simulink model "Hybrid_Series"  (R2017b)
settings: Solver=VariableStepAuto  StartTime=0.0  StopTime=20  RelTol=1e-3  AbsTol=1e-3  EnableMultiTasking=on
model workspace (MATLAB code in the model file):
  | v0                 = 15; % Initial vehicle speed
  | wheel_radius = 0.3; % Wheel radius
  | k                   = 1e-2; % Motor losses (W/(N*M)^2)
  | t_torque        = 0.02; % Electric motor time constant
  | rpm0             = 2000; % Engine initial speed demand
values from neighbouring files (symbols this model uses):
  HEV_Param =     [DataWorkSpace.mat]
libraries: fl_lib x83, nesl_utility x27, sdl_lib x5, elec_lib x2
(part 1 of 2)
CloseFcn:
  | try,close(h1_sdl_hybrid_series),end
  | clear h1_sdl_hybrid_series
  | try,close(h2_sdl_hybrid_series),end
  | clear h2_sdl_hybrid_series
  | 
  | 
  | clear simlog_sdl_hybrid_series
Description:
  | Series Hybrid Transmission
  | 
  | Copyright 2008-2017 The MathWorks, Inc.
settings Model: FPTRunName=Active  Creator=MathWorks  LastModifiedBy=Charlie
settings DataIOCC: LimitDataPoints=on  MaxDataPoints=15000  SaveFormat=Array  SignalLoggingSaveFormat=ModelDataLogs  SignalLoggingName=logsout_sdl_hybrid_series
settings OptimizationCC: ExpressionDepthLimit=2147483647  LifeSpan=inf
settings DebuggingCC: UnderspecifiedInitializationDetection=Classic  MergeDetectMultiDrivingBlocksExec=none  FcnCallInpInsideContextMsg=warning  StateNameClashWarn=warning  SFUnexpectedBacktrackingDiag=warning  SFNoUnconditionalDefaultTransitionDiag=warning  SFExecutionAtInitializationDiag=none
settings HardwareCC: ProdBitPerPointer=32  ProdBitPerSizeT=32  ProdBitPerPtrDiffT=32  ProdLargestAtomicFloat=None  ProdIntDivRoundTo=Undefined  ProdEndianess=Unspecified  ProdWordSize=32  ProdHWDeviceType=32-bit Generic
settings ModelReferenceCC: PropagateSignalLabelsOutOfModel=off
settings CodeAppCC: StateflowObjectComments=on
settings GRTTargetCC: TargetLangStandard=C89/C90 (ANSI)  GeneratePreprocessorConditionals=Disable all  CombineOutputUpdateFcns=off  GRTInterface=on
settings ConfigComp: CovMetricSettings=dw  CovHtmlReporting=on  CovSaveCumulativeToWorkspaceVar=on  CovSaveSingleToWorkspaceVar=on  CovShowResultsExplorer=off  CovExternalEMLEnable=off
settings SimscapeCC: SimscapeLogType=all  SimscapeLogSimulationStatistics=on  SimscapeLogOpenViewer=on  SimscapeLogName=simlog_sdl_hybrid_series  SimscapeLogDataHistory=10000

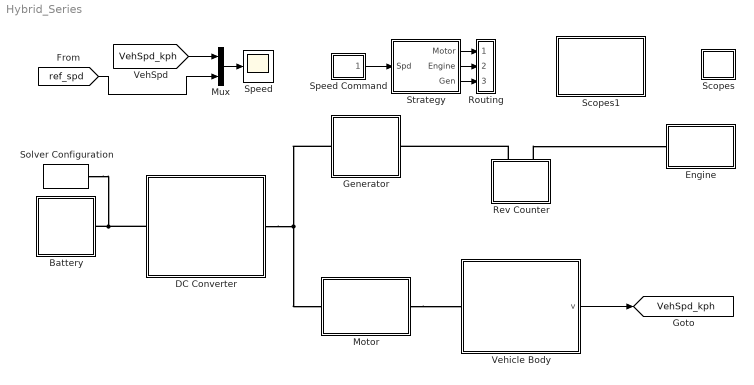
== system Hybrid_Series ==
  Battery : Subsystem
      mask Display:
      | % Plot points to set plot range
      | color('white');plot(1.5, 2.5);plot(-1.5, -2)
      | color('black');
      | % Battery icon
      | plot([0 0], [2.5 1.3])
      | plot([0 0], [-0.6 -1.6])
      | patch([-1 1 1 -1]*0.4, [1 1 -1 -1]*0.15+0.7,[0;0;0]);
      | patch([-1 1 1 -1]*0.4, [1 1 -1 -1]*0.15-0.6,[0;0;0]);
      | patch([-1 1 1 -1]*0.8, [1 1 -1 -1]*0.15+1.3,[0;0;0]);
      | patch([-1 1 1 -1]*0.8, [1 1 -1 -1]*0.15+0.0,[0;0;0]);
  DC Converter : Subsystem  mask{Vout=HEV_Param.DCDCConv.Output_Voltage, RLoadLoss=HEV_Param.DCDCConv.Resistance_Losses, Kp=HEV_Param.DCDCConv.Kp, Ki=HEV_Param.DCDCConv.Ki}
      mask prompts: Vout "Output Voltage (V)"; RLoadLoss "Resistance, Load Dependent Losses (Ohm)"; Kp "Proportional Gain"; Ki "Integral Gain"
      mask Display: image('D:\Matlab\Powertrain\Simscape\DC.jpg');
  Engine : Subsystem
      mask Display:
      | patch([0 374 374 0 0],[183 40 40 183 183],[1 1 1]);
      | plot([200.294537656123;201.704177092068;202.879954177142;203.81054553527;204.486989062962;204.902770239264;205.053884864158;204.938877621199;204.558856093007;203.917480094638;203.02092642757;201.877829393721;200.499197642409;198.898308151034;197.090578360535;195.093417696999;192.926059909376;191.349221415216], [79.0962651705123;81.4129472419303;83.856642682368;86.4038173688741;89.0299406167901;91.7097214236537;94.4173520353776;97.1267564890293;99.8118417386092;102.446748945347;105.006102512455;107.465254465996;109.80052182835;111.989414698229;114.010852840726;115.845368701499;117.475294889959;118.468271604945])
      | plot([180.070315486255;177.215173525063;174.340173090774;171.473002009205;168.641272705228;165.872256280019;163.192619875453;160.628169854943;158.203603274058;155.942270034374;153.865948011161;151.994633320535;150.346347745932;148.936965178479;147.780058742747;146.886770080143;146.265702048809;145.922835873396;145.861473542603;146.08220600922;146.58290749893;147.358755982674;148.402279615432;149.703428694174;151.249672441989;153.026119686324;155.015662269112;157.199139807684;159.555524219735;162.062122235246;164.694793945081;167.42818528151;170.23597219174;173.091114152932;175.966114587221;178.83328566879;181.665014972767;184.434031397976;185.486929355725], [123.25590763568;123.598773811093;123.660136141886;123.439403675268;122.938702185559;122.162853701815;121.119330069056;119.818180990315;118.2719372425;116.495489998164;114.505947415377;112.322469876805;109.966085464754;107.459487449243;104.826815739408;102.093424402979;99.2856374927491;96.4304955315569;93.5554950972677;90.688324015699;87.8565947117214;85.0875782865128;82.4079418819464;79.8434918614364;77.4189252805513;75.1575920408679;73.081270017655;71.2099553270291;69.5616697524256;68.1522871849724;66.9953807492411;66.1020920866371;65.4810240553025;65.1381578798894;65.0767955490969;65.2975280157144;65.7982295054238;66.5740779891678;66.9481130562871])
      | plot([182.088349247351;182.056804583223;181.962474383197;181.806267098667;181.589687091173;181.314820144583;180.98431337785;180.601349751811;180.169617415534;179.693274187426;179.176907513169;178.625490286111;178.044332955585;177.439032384376;176.815417947876;176.17949539401;175.537389004603;174.895282615196;174.25936006133;173.63574562483;173.030445053621;172.449287723095;171.897870496037;171.38150382178;170.905160593672;170.473428257395;170.090464631356;169.759957864623;169.485090918033;169.268510910539;169.112303626009;169.017973425983;168.986428761855;169.017973425983;169.112303626009;169.268510910539;169.485090918033;169.759957864623;170.090464631356;170.473428257395;170.905160593672;171.38150382178;171.897870496037;172.449287723095;173.030445053621;173.63574562483;174.25936006133;174.895282615196;175.537389004603;176.17949539401;176.815417947876;177.439032384376;178.044332955585;178.625490286111;179.176907513169;179.693274187426;180.169617415534;180.601349751811;180.98431337785;181.314820144583;181.589687091173;181.806267098667;181.962474383197;182.056804583223;182.088349247351;182.088349247351], [94.3432759959251;93.7073437064164;93.0775357924916;92.4599176486499;91.8604372752408;91.2848679959696;90.7387528576339;90.2273512475527;89.7555882427917;89.3280071789786;88.9487258954975;88.6213970784445;88.3491730832641;88.1346755758426;87.9799702844327;87.8865471055612;87.8553057555109;87.8865471055612;87.9799702844327;88.1346755758426;88.3491730832641;88.6213970784445;88.9487258954975;89.3280071789786;89.7555882427917;90.2273512475527;90.7387528576339;91.2848679959696;91.8604372752408;92.4599176486499;93.0775357924916;93.7073437064164;94.3432759959251;94.9792082854337;95.6090161993586;96.2266343432003;96.8261147166093;97.4016839958805;97.9477991342162;98.4592007442974;98.9309637490584;99.3585448128716;99.7378260963527;100.065154913406;100.337378908586;100.551876416008;100.706581707417;100.800004886289;100.831246236339;100.800004886289;100.706581707417;100.551876416008;100.337378908586;100.065154913406;99.7378260963526;99.3585448128716;98.9309637490584;98.4592007442974;97.9477991342162;97.4016839958805;96.8261147166093;96.2266343432003;95.6090161993586;94.9792082854338;94.3432759959251;94.3432759959251])
      | plot([201.615249970928;201.583705306799;201.489375106774;201.333167822243;201.11658781475;200.84172086816;200.511214101427;200.128250475388;199.69651813911;199.220174911002;198.703808236745;198.152391009688;197.571233679162;196.965933107953;196.342318671452;195.706396117586;195.06428972818;194.422183338773;193.786260784907;193.162646348407;192.557345777197;191.976188446671;191.424771219614;190.908404545357;190.432061317249;190.000328980971;189.617365354932;189.286858588199;189.011991641609;188.795411634116;188.639204349585;188.54487414956;188.513329485431;188.54487414956;188.639204349585;188.795411634116;189.011991641609;189.286858588199;189.617365354932;190.000328980971;190.432061317249;190.908404545357;191.424771219614;191.976188446671;192.557345777197;193.162646348407;193.786260784907;194.422183338773;195.06428972818;195.706396117586;196.342318671452;196.965933107953;197.571233679162;198.152391009688;198.703808236745;199.220174911002;199.69651813911;200.128250475388;200.511214101427;200.84172086816;201.11658781475;201.333167822243;201.489375106774;201.583705306799;201.615249970928;201.615249970928], [74.7533852700144;74.1174529805057;73.487645066581;72.8700269227392;72.2705465493302;71.694977270059;71.1488621317233;70.6374605216421;70.165697516881;69.7381164530679;69.3588351695868;69.0315063525339;68.7592823573535;68.5447848499319;68.390079558522;68.2966563796505;68.2654150296003;68.2966563796505;68.390079558522;68.5447848499319;68.7592823573535;69.0315063525339;69.3588351695868;69.7381164530679;70.165697516881;70.6374605216421;71.1488621317233;71.694977270059;72.2705465493302;72.8700269227392;73.487645066581;74.1174529805057;74.7533852700144;75.3893175595231;76.0191254734479;76.6367436172896;77.2362239906986;77.8117932699698;78.3579084083055;78.8693100183867;79.3410730231478;79.7686540869609;80.147935370442;80.4752641874949;80.7474881826754;80.9619856900969;81.1166909815068;81.2101141603783;81.2413555104285;81.2101141603783;81.1166909815068;80.9619856900969;80.7474881826753;80.4752641874949;80.147935370442;79.7686540869609;79.3410730231478;78.8693100183867;78.3579084083055;77.8117932699698;77.2362239906986;76.6367436172896;76.0191254734479;75.3893175595231;74.7533852700145;74.7533852700144])
      | plot([201.615249970928;201.583705306799;201.489375106774;201.333167822243;201.11658781475;200.84172086816;200.511214101427;200.128250475388;199.69651813911;199.220174911002;198.703808236745;198.152391009688;197.571233679162;196.965933107953;196.342318671452;195.706396117586;195.06428972818;194.422183338773;193.786260784907;193.162646348407;192.557345777197;191.976188446671;191.424771219614;190.908404545357;190.432061317249;190.000328980971;189.617365354932;189.286858588199;189.011991641609;188.795411634116;188.639204349585;188.54487414956;188.513329485431;188.54487414956;188.639204349585;188.795411634116;189.011991641609;189.286858588199;189.617365354932;190.000328980971;190.432061317249;190.908404545357;191.424771219614;191.976188446671;192.557345777197;193.162646348407;193.786260784907;194.422183338773;195.06428972818;195.706396117586;196.342318671452;196.965933107953;197.571233679162;198.152391009688;198.703808236745;199.220174911002;199.69651813911;200.128250475388;200.511214101427;200.84172086816;201.11658781475;201.333167822243;201.489375106774;201.583705306799;201.615249970928;201.615249970928], [74.7533852700144;74.1174529805057;73.487645066581;72.8700269227392;72.2705465493302;71.694977270059;71.1488621317233;70.6374605216421;70.165697516881;69.7381164530679;69.3588351695868;69.0315063525339;68.7592823573535;68.5447848499319;68.390079558522;68.2966563796505;68.2654150296003;68.2966563796505;68.390079558522;68.5447848499319;68.7592823573535;69.0315063525339;69.3588351695868;69.7381164530679;70.165697516881;70.6374605216421;71.1488621317233;71.694977270059;72.2705465493302;72.8700269227392;73.487645066581;74.1174529805057;74.7533852700144;75.3893175595231;76.0191254734479;76.6367436172896;77.2362239906986;77.8117932699698;78.3579084083055;78.8693100183867;79.3410730231478;79.7686540869609;80.147935370442;80.4752641874949;80.7474881826754;80.9619856900969;81.1166909815068;81.2101141603783;81.2413555104285;81.2101141603783;81.1166909815068;80.9619856900969;80.7474881826753;80.4752641874949;80.147935370442;79.7686540869609;79.3410730231478;78.8693100183867;78.3579084083055;77.8117932699698;77.2362239906986;76.6367436172896;76.0191254734479;75.3893175595231;74.7533852700145;74.7533852700144])
      | plot([142.90856779553;142.90856779553;208.103220211342;208.103220211342], [139.948037685826;218.181620584801;218.181620584801;139.948037685826])
      | plot([142.90856779553;208.103220211342], [179.064829135314;179.064829135314])
      | plot([149.459528038278;149.459528038278], [179.064829135314;172.576858894899])
      | plot([201.615249970928;201.615249970928], [179.064829135314;172.576858894899])
      | plot([142.90856779553;208.103220211342;208.103220211342;142.90856779553;142.90856779553], [179.064829135314;179.064829135314;152.986968168989;152.986968168989;179.064829135314])
      | plot([142.90856779553;208.103220211342], [192.103759618476;192.103759618476])
      | plot([180.639579193667;200.229469919577], [99.0045361686498;79.4776354450732])
      | plot([173.332738922909;192.92262964882], [87.8553057555109;68.3284050319344])
      | plot([183.663099305704;200.481429928914], [153.553878189996;76.9580353517085])
      | plot([184.544959338382;174.970478983596], [95.0361660216004;153.553878189996])
      | plot([183.474129298702;186.749609420076;206.654450157657;201.615249970928;197.961829835549], [76.9580353517085;62.0923948008567;67.8874750155956;88.1702557671815;87.7923157531768])
      | plot([164.199188584462;187.694459455088], [94.7842060122639;95.1621460262686])
      | plot([175.537389004603;175.285428995267], [106.50034644641;81.9342455361038])
      | plot([142.90856779553;208.103220211342], [172.576858894899;172.576858894899])
      | plot([297.86397353746;317.389525743201], [71.0999651346356;71.0999651346356]+60)
      | plot([269.518472487107;297.86397353746;297.86397353746;269.518472487107;269.518472487107], [85.2727156598121;85.2727156598121;56.927214609459;56.927214609459;85.2727156598121]+60)
      | plot([258.180272066966;269.518472487107;269.518472487107;258.180272066966], [42.7544640842825;42.7544640842825;99.4454661849886;99.4454661849886]+60)
      | plot([108.893966535106;108.245686045801;107.603648851995;106.974038122836;106.362917353826;105.776171972045;105.219452656266;104.698120917834;104.217197466378;103.781313857637;103.394667889039;103.060983172626;102.783473274627;102.564810767061;102.40710148941;102.31186426823;102.280016290024;102.280016290024;102.31186426823;102.40710148941;102.564810767061;102.783473274627;103.060983172626;103.394667889039;103.781313857637;104.217197466378;104.698120917834;105.219452656266;105.776171972045;106.362917353826;106.974038122836;107.603648851995;108.245686045801;108.893966535106;249.67662175186;250.324902241165;250.966939434972;251.596550164131;252.20767093314;252.794416314921;253.3511356307;253.872467369133;254.353390820588;254.78927442933;255.175920397927;255.50960511434;255.787115012339;256.005777519905;256.163486797556;256.258724018736;256.290571996942;256.290571996942;256.258724018736;256.163486797556;256.005777519905;255.787115012339;255.50960511434;255.175920397927;254.78927442933;254.353390820588;253.872467369133;253.3511356307;252.794416314921;252.20767093314;251.596550164131;250.966939434972;250.324902241165;249.67662175186;108.893966535106], [233.173241140321;233.141393162114;233.046155940935;232.888446663284;232.669784155718;232.392274257719;232.058589541306;231.671943572708;231.236059963967;230.755136512511;230.233804774079;229.6770854583;229.090340076519;228.479219307509;227.84960857835;227.207571384544;226.559290895239;46.5338642243296;45.8855837350246;45.2435465412178;44.6139358120588;44.0028150430496;43.4160696612682;42.8593503454891;42.3380186070568;41.8570951556014;41.4212115468599;41.0345655782626;40.7008808618494;40.42337096385;40.2047084562844;40.0469991786335;39.9517619574538;39.9199139792472;39.9199139792472;39.9517619574538;40.0469991786335;40.2047084562844;40.42337096385;40.7008808618494;41.0345655782626;41.4212115468599;41.8570951556014;42.3380186070568;42.8593503454891;43.4160696612682;44.0028150430496;44.6139358120588;45.2435465412178;45.8855837350246;46.5338642243296;226.559290895239;227.207571384544;227.84960857835;228.479219307509;229.090340076519;229.6770854583;230.233804774079;230.755136512511;231.236059963967;231.671943572708;232.058589541306;232.392274257719;232.669784155718;232.888446663284;233.046155940935;233.141393162114;233.173241140321;233.173241140321])
  Generator : Subsystem
      mask Display: image('D:\Matlab\Powertrain\Simscape\Yanan_400_hertz_brushless_generator_alternator_3984_3.jpg');
  Motor : Subsystem
      mask Display: image('D:\Matlab\Powertrain\Simscape\IM2014100062CO_300dpi.jpg');
  Mux : Mux  Inputs=2
  Rev Counter : Subsystem
      mask Display: image('D:\Matlab\Powertrain\Simscape\Rev-counter.jpg');
  Routing : Subsystem
  Scopes : Subsystem
  Scopes1 : Subsystem  mask(Data Acquisition){}
      mask Display: image('D:\Matlab\Powertrain\Plot\Fuel_Tank.jpg');
  Solver Configuration : nesl_utility/Solver Configuration  PhysicalDomain=network_engine_domain  SubClassName=solver  LeftPortType=input  RightPortType=generic  Accelerate=off  Tones=[]  Harmonics=[]  SimulateNoise=off  Profile=off  UseLocalSampling=off  EnableSwitchedLinearOptims=on  FrequencyDomain=off  UseCCode=off  RelTol=0.001  AbsTol=1e-06  MinStep=1e-09  ToWorkspace=off  RevertToSquareIcSolve=off  NumHomotopyIterations=100  PhasorMode=off  PhasorModeNumHarmonics=1  DoDC=off  ResidualTolerance=1e-9  UseLocalSolver=off  LocalSolverChoice=NE_BACKWARD_EULER_ADVANCER  LocalSolverSampleTime=0.005  DoFixedCost=off  MaxNonlinIter=3  MaxModeIter=2  LinearAlgebra=Sparse  DelaysMemoryBudget=1024  AutomaticFiltering=on  FilteringTimeConstant=0.001
  Speed : Scope
  Speed Command : Subsystem
  Strategy : Subsystem
  Vehicle Body : Subsystem
      mask Display: image('D:\Matlab\Powertrain\Simscape\smart_fortw.jpg');
  tag scope: VehSpd_kph=global
  wires:
  Speed Command/1(Spd) -> Strategy/1(Spd)
  Strategy/1(Motor) -> Routing/1(M)
  Strategy/2(Engine) -> Routing/2(E)
  Strategy/3(Gen) -> Routing/3(G)
  Mux/1 -> Speed/1
  [ref_spd] -> Mux/2
  Vehicle Body/1(v) -> [VehSpd_kph]
  [VehSpd_kph] -> Mux/1
  connections:
  Motor/LConn1 -- Vehicle Body/LConn1
  Generator/RConn1 -- DC Converter/RConn1 -- Motor/RConn1
  Solver Configuration/RConn1 -- DC Converter/LConn1 -- Battery/LConn1
  Rev Counter/LConn2 -- Engine/RConn1
  Rev Counter/LConn1 -- Generator/LConn1

== system Hybrid_Series/Battery ==
  Calculations : Subsystem
  Current Sensor : fl_lib/Electrical/Electrical Sensors/Current Sensor
  DC Voltage Source : fl_lib/Electrical/Electrical Sources/DC Voltage Source  v0=201.6 V
  Electrical Reference : fl_lib/Electrical/Electrical Elements/Electrical Reference
  Internal Resistance : fl_lib/Electrical/Electrical Elements/Resistor  R=0.05 Ohm  i_specify=off  i_priority=High  i=0 A  i_nominal_specify=off  i_nominal_unit=A  i_nominal_value=1  v_specify=off  v_priority=High  v=0 V  v_nominal_specify=off  v_nominal_unit=V  v_nominal_value=1
  Voltage Sensor : fl_lib/Electrical/Electrical Sensors/Voltage Sensor
  V : PMIOPort  Port=1  Side=Left
  connections:
  DC Voltage Source/LConn1 -- Internal Resistance/LConn1
  Internal Resistance/RConn1 -- V/RConn1 -- Voltage Sensor/LConn1
  Current Sensor/RConn2 -- DC Voltage Source/RConn1
  Voltage Sensor/RConn1 -- Calculations/LConn1
  Current Sensor/RConn1 -- Calculations/LConn2
  Electrical Reference/LConn1 -- Current Sensor/LConn1 -- Voltage Sensor/RConn2

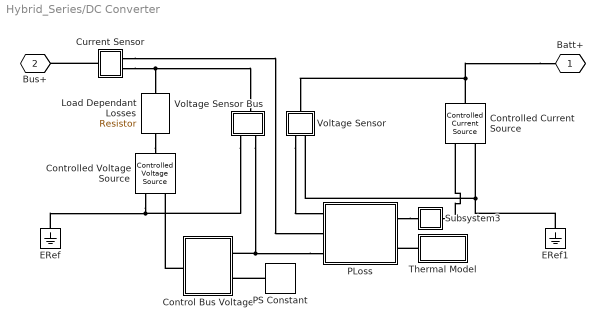
== system Hybrid_Series/DC Converter ==
  Control Bus Voltage : Subsystem
  Controlled Current Source : fl_lib/Electrical/Electrical Sources/Controlled Current Source
  Controlled Voltage Source : fl_lib/Electrical/Electrical Sources/Controlled Voltage Source
  Current Sensor : Subsystem
  ERef : fl_lib/Electrical/Electrical Elements/Electrical Reference
  ERef1 : fl_lib/Electrical/Electrical Elements/Electrical Reference
  Load Dependant Losses : fl_lib/Electrical/Electrical Elements/Resistor  R=RLoadLoss Ohm  i_specify=off  i_priority=High  i=0 A  i_nominal_specify=off  i_nominal_unit=A  i_nominal_value=1  v_specify=off  v_priority=High  v=0 V  v_nominal_specify=off  v_nominal_unit=V  v_nominal_value=1
  PLoss : Subsystem
  PS Constant : fl_lib/Physical Signals/Sources/PS Constant  constant=Vout
  Subsystem3 : Subsystem
      mask Display: disp('S')
  Thermal Model : Subsystem
  Voltage Sensor : Subsystem
  Voltage Sensor Bus : Subsystem
  " Batt+" : PMIOPort  Tag=PMCPort  Port=1  Side=Left
  " Bus+" : PMIOPort  Tag=PMCPort  Port=2  Side=Right
  connections:
  Thermal Model/LConn1 -- PLoss/RConn2
  PLoss/LConn3 -- Control Bus Voltage/LConn1 -- Voltage Sensor Bus/RConn2
  Subsystem3/LConn1 -- Controlled Current Source/RConn1
  PS Constant/RConn1 -- Control Bus Voltage/LConn2
  Control Bus Voltage/RConn1 -- Controlled Voltage Source/RConn1
  " Batt+"/RConn1 -- Controlled Current Source/LConn1 -- Voltage Sensor/LConn1
  Controlled Current Source/RConn2 -- ERef1/LConn1 -- Voltage Sensor/RConn2
  Load Dependant Losses/RConn1 -- Controlled Voltage Source/LConn1
  Controlled Voltage Source/RConn2 -- ERef/LConn1 -- Voltage Sensor Bus/RConn1
  Current Sensor/LConn1 -- " Bus+"/RConn1
  Current Sensor/RConn2 -- Load Dependant Losses/LConn1 -- Voltage Sensor Bus/LConn1
  Voltage Sensor/RConn1 -- PLoss/LConn1
  Current Sensor/RConn1 -- PLoss/LConn2
  PLoss/RConn1 -- Subsystem3/RConn1

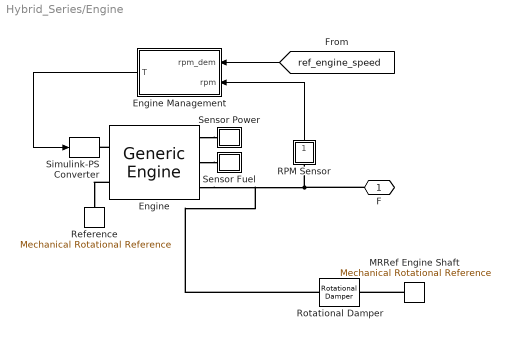
== system Hybrid_Series/Engine ==
  Engine : sdl_lib/Engines/Generic Engine  model_parameterization=1  engine_type=1  P_max=52 kW  w_P_max=6000 rpm  w_max=7000 rpm  w_min=500 rpm  w_tab=[ 500 1000 2e+3 3e+3 4e+3 5e+3 6e+3 7e+3 ] rpm  trq_tab=[ 40 41 42 46 49 42 41 40 ] N*m  pwr_tab=[ 2e+4 4e+4 7.8e+4 1.2e+5 1.45e+5 1.48e+5 1.25e+5 6e+4 ] W  interp_method=1  model_inertia=1  inertia=HEV_Param.ICE.Shaft_Inertia kg*m^2  initial_velocity=2000 rpm  model_time_constant=1  time_constant=0.4 s  T0=0  w_thr=100 rpm  idle_speed=1  idle_speed_reference=800 rpm  tau_controller=1 s  idle_w_thr=1 rpm  redline=0  redline_speed=7000 rpm  tau_redline=1 s  redline_w_thr=1 rpm  fc_model=1  fc_per_rev=6.2 mg/rev  displaced_volume=400 cm^3  rev_per_cycle=2  fc_w_tab=[ 1000 2e+3 3e+3 4e+3 5e+3 6e+3 ] rpm  fc_trq_tab=[ 0 80 160 200 240 320 360 400 ] N*m  fc_tab=[ 0.5 0.9 1.4 1.6 1.9 2.7 3.4 4.4; 1 1.7 2.7 3.1 3.6 5 6 7.4; 1.4 2.7 4 4.8 5.6 7.5 8.5 10.5; 2 3.6 5.8 6.7 8 10.4 11.7 13.3; 2.5 4.8 7.9 9.4 10.8 14 16.2 18.6; 3.1 6 10.3 11.9 13.8 18.4 22 26.5 ] g/s  bmep_tab=[ 0 250 500 625 750 1000 1.15e+3 1.25e+3 ] kPa  bsfc_tab=[ 410 380 300 280 270 290 320 380; 410 370 290 270 260 270 285 320; 415 380 290 275 265 270 270 300; 420 390 310 290 285 280 280 285; 430 410 340 320 310 300 310 320; 450 430 370 340 330 330 350 380 ] g/hr/kW  fc_interp_method=1
      settings: SourceProductName=Simscape Driveline  SourceProductBaseCode=LD
  Engine Management : Subsystem
  MRRef Engine Shaft : fl_lib/Mechanical/Rotational Elements/Mechanical Rotational Reference
  RPM Sensor : Subsystem
      mask Display: disp('S');
  Reference : fl_lib/Mechanical/Rotational Elements/Mechanical Rotational Reference
  Rotational Damper : fl_lib/Mechanical/Rotational Elements/Rotational Damper  D=HEV_Param.ICE.Friction N*m/(rad/s)  w_specify=off  w_priority=High  w=0 rad/s  w_nominal_specify=off  w_nominal_unit=rad/s  w_nominal_value=1  t_specify=off  t_priority=High  t=0 N*m  t_nominal_specify=off  t_nominal_unit=N*m  t_nominal_value=1
  Sensor Fuel : Subsystem
  Sensor Power : Subsystem
  Simulink-PS Converter : nesl_utility/Simulink-PS Converter  PhysicalDomain=network_engine_domain  SubClassName=ps_input  LeftPortType=input  RightPortType=output  PseudoPeriodic=off  Frequencies=[]  NoiseDistribution=none  NoiseParameters=[]  Unit=1  AffineConversion=off  FilteringAndDerivatives=zero  SimscapeFilterOrder=1  InputFilterTimeConstant=.001  UdotUserProvided=0
  F : PMIOPort  Port=1  Side=Right
  wires:
  RPM Sensor/1(rpm) -> Engine Management/2(rpm)
  [ref_engine_speed] -> Engine Management/1(rpm_dem)
  Engine Management/1(T) -> Simulink-PS Converter/1
  connections:
  F/RConn1 -- Rotational Damper/LConn1 -- Engine/RConn3 -- RPM Sensor/LConn1
  Engine/LConn2 -- Reference/LConn1
  Engine/LConn1 -- Simulink-PS Converter/RConn1
  Engine/RConn1 -- Sensor Power/LConn1
  Engine/RConn2 -- Sensor Fuel/LConn1
  MRRef Engine Shaft/LConn1 -- Rotational Damper/RConn1

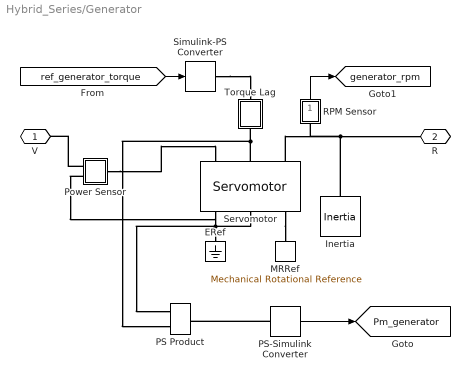
== system Hybrid_Series/Generator ==
  ERef : fl_lib/Electrical/Electrical Elements/Electrical Reference
  Inertia : fl_lib/Mechanical/Rotational Elements/Inertia  inertia=HEV_Param.Generator.Shaft_Inertia kg*m^2  w_specify=on  w_priority=High  w=0 rad/s  w_nominal_specify=off  w_nominal_unit=rad/s  w_nominal_value=1  t_specify=off  t_priority=High  t=0 N*m  t_nominal_specify=off  t_nominal_unit=N*m  t_nominal_value=1
  MRRef : fl_lib/Mechanical/Rotational Elements/Mechanical Rotational Reference
  PS Product : fl_lib/Physical Signals/Functions/PS Product
      settings: SourceProductName=Simscape
  PS-Simulink Converter : nesl_utility/PS-Simulink Converter  PhysicalDomain=network_engine_domain  SubClassName=ps_output  LeftPortType=input  RightPortType=output  PseudoPeriodic=off  Frequencies=[]  Unit=1  AffineConversion=off
  Power Sensor : Subsystem  AncestorBlock=HEV_Electrical_Lib/System Level/Synchronous Generator & Drive/Power Sensor
      mask Display: disp('S')
  RPM Sensor : Subsystem
      mask Display: disp('S')
  Servomotor : elec_lib/Actuators & Drivers/Rotational Actuators/Servomotor  torque_speed_param=1  w_t=HEV_Param.Generator.TorqSpdLUT.SpeedRPM rpm  T_t=HEV_Param.Generator.TorqSpdLUT.TorqueNm N*m  torque_max=0.1 N*m  power_max=30 W  Tc=HEV_Param.Generator.TorqueControl_TimeConst s  losses_param=1  eff=90  w_eff=2000 rpm  T_eff=200 N*m  Piron=0 W  Pbase=HEV_Param.Generator.TorqIndep_Elec_Loss W  w_eff_vec=[-8000 -4000 0 4000 8000] rpm  T_eff_vec=[0 0.03 0.06 0.09] N*m  losses_mat=[1.49 1.67 2.21 3.10; 0.42 0.69 1.14 2.03; 0.06 0.24 0.78 1.68; 0.42 0.69 1.14 2.03; 1.49 1.67 2.21 3.10] W  efficiency_mat=[95 95 95 95; 95 95 95 95; 95 95 95 95; 95 95 95 95; 95 95 95 95]  Res=HEV_Param.Generator.Series_Resistance Ohm  J=0 kg*m^2  lam=HEV_Param.Generator.Damping N*m/(rad/s)  speed0=0 rpm  faulted_specify=off  faulted_priority=None  faulted=0  faulted_nominal_specify=off  faulted_nominal_unit=1  faulted_nominal_value=1  alpha=0.00393 1/K  Tmeas=25 degC  Tmeas2=125 degC  losses_mat_T2=[1.49 1.74 2.49 3.74;0.42 0.67 1.42 2.67;0.06 0.31 1.06 2.31;0.42 0.67 1.42 2.67;1.49 1.74 2.49 3.74] W  efficiency_mat_T2=[95 95 95 95; 95 95 95 95; 95 95 95 95; 95 95 95 95; 95 95 95 95]  thermal_mass=100 J/K  initial_temperature=25 degC  fault_condition=1  fault_threshold=0.5
      settings: SourceProductName=Simscape Electronics  SourceProductBaseCode=SN
  Simulink-PS Converter : nesl_utility/Simulink-PS Converter  PhysicalDomain=network_engine_domain  SubClassName=ps_input  LeftPortType=input  RightPortType=output  PseudoPeriodic=off  Frequencies=[]  NoiseDistribution=none  NoiseParameters=[]  Unit=N*m  AffineConversion=off  FilteringAndDerivatives=zero  SimscapeFilterOrder=1  InputFilterTimeConstant=.001  UdotUserProvided=0
  Torque Lag : Subsystem
  V : PMIOPort  Port=1  Side=Right
  R : PMIOPort  Port=2  Side=Left
  tag scope: Pm_generator=global, generator_rpm=global
  wires:
  [ref_generator_torque] -> Simulink-PS Converter/1
  RPM Sensor/1(rpm) -> [generator_rpm]
  PS-Simulink Converter/1 -> [Pm_generator]
  connections:
  Servomotor/RConn1 -- Power Sensor/LConn2 -- ERef/LConn1
  Servomotor/RConn3 -- MRRef/LConn1
  Servomotor/LConn3 -- RPM Sensor/LConn1 -- Inertia/LConn1 -- R/RConn1
  Simulink-PS Converter/RConn1 -- Torque Lag/LConn1
  Torque Lag/RConn1 -- Servomotor/LConn2 -- PS Product/LConn2
  Servomotor/RConn2 -- PS Product/LConn1
  PS-Simulink Converter/LConn1 -- PS Product/RConn1
  Power Sensor/LConn1 -- V/RConn1
  Power Sensor/RConn1 -- Servomotor/LConn1

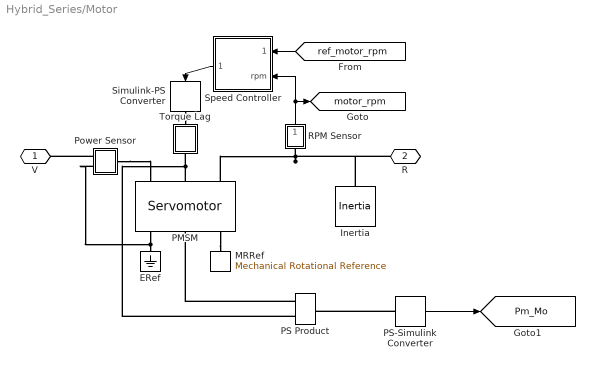
== system Hybrid_Series/Motor ==
  ERef : fl_lib/Electrical/Electrical Elements/Electrical Reference
  Inertia : fl_lib/Mechanical/Rotational Elements/Inertia  inertia=HEV_Param.Motor.Shaft_Inertia kg*m^2  w_specify=on  w_priority=High  w=0 rad/s  w_nominal_specify=off  w_nominal_unit=rad/s  w_nominal_value=1  t_specify=off  t_priority=High  t=0 N*m  t_nominal_specify=off  t_nominal_unit=N*m  t_nominal_value=1
  MRRef : fl_lib/Mechanical/Rotational Elements/Mechanical Rotational Reference
  PMSM : elec_lib/Actuators & Drivers/Rotational Actuators/Servomotor  torque_speed_param=1  w_t=HEV_Param.Motor.TorqSpdLUT.SpeedRPM rpm  T_t=HEV_Param.Motor.TorqSpdLUT.TorqueNm N*m  torque_max=0.1 N*m  power_max=30 W  Tc=HEV_Param.Motor.TorqueControl_TimeConst s  losses_param=1  eff=HEV_Param.Motor.Efficiency  w_eff=2000 rpm  T_eff=200 N*m  Piron=0 W  Pbase=0 W  w_eff_vec=[-8000 -4000 0 4000 8000] rpm  T_eff_vec=[0 0.03 0.06 0.09] N*m  losses_mat=[1.49 1.67 2.21 3.10; 0.42 0.69 1.14 2.03; 0.06 0.24 0.78 1.68; 0.42 0.69 1.14 2.03; 1.49 1.67 2.21 3.10] W  efficiency_mat=[95 95 95 95; 95 95 95 95; 95 95 95 95; 95 95 95 95; 95 95 95 95]  Res=HEV_Param.Motor.Series_Resistance Ohm  J=0 kg*m^2  lam=HEV_Param.Motor.Damping N*m/(rad/s)  speed0=0 rpm  faulted_specify=off  faulted_priority=None  faulted=0  faulted_nominal_specify=off  faulted_nominal_unit=1  faulted_nominal_value=1  alpha=0.00393 1/K  Tmeas=25 degC  Tmeas2=125 degC  losses_mat_T2=[1.49 1.74 2.49 3.74;0.42 0.67 1.42 2.67;0.06 0.31 1.06 2.31;0.42 0.67 1.42 2.67;1.49 1.74 2.49 3.74] W  efficiency_mat_T2=[95 95 95 95; 95 95 95 95; 95 95 95 95; 95 95 95 95; 95 95 95 95]  thermal_mass=100 J/K  initial_temperature=25 degC  fault_condition=1  fault_threshold=0.5
      settings: SourceProductName=Simscape Electronics  SourceProductBaseCode=SN
  PS Product : fl_lib/Physical Signals/Functions/PS Product
      settings: SourceProductName=Simscape
  PS-Simulink Converter : nesl_utility/PS-Simulink Converter  PhysicalDomain=network_engine_domain  SubClassName=ps_output  LeftPortType=input  RightPortType=output  PseudoPeriodic=off  Frequencies=[]  Unit=1  AffineConversion=off
  Power Sensor : Subsystem  AncestorBlock=HEV_Electrical_Lib/System Level/Synchronous Generator & Drive/Power Sensor
      mask Display: disp('S')
  RPM Sensor : Subsystem
      mask Display: disp('S')
  Simulink-PS Converter : nesl_utility/Simulink-PS Converter  PhysicalDomain=network_engine_domain  SubClassName=ps_input  LeftPortType=input  RightPortType=output  PseudoPeriodic=off  Frequencies=[]  NoiseDistribution=none  NoiseParameters=[]  Unit=N*m  AffineConversion=off  FilteringAndDerivatives=zero  SimscapeFilterOrder=1  InputFilterTimeConstant=.001  UdotUserProvided=0
  Speed Controller : Subsystem
  Torque Lag : Subsystem
  V : PMIOPort  Port=1  Side=Right
  R : PMIOPort  Port=2  Side=Left
  tag scope: Pm_Mo=global, motor_rpm=global
  wires:
  Speed Controller/1(T_ref) -> Simulink-PS Converter/1
  [ref_motor_rpm] -> Speed Controller/1(rpm_ref)
  RPM Sensor/1(rpm) -> [motor_rpm], Speed Controller/2(rpm)
  PS-Simulink Converter/1 -> [Pm_Mo]
  connections:
  RPM Sensor/LConn1 -- Inertia/LConn1 -- R/RConn1 -- PMSM/LConn3
  PMSM/LConn2 -- PS Product/LConn2 -- Torque Lag/RConn1
  PMSM/RConn1 -- Power Sensor/LConn2 -- ERef/LConn1
  PMSM/RConn3 -- MRRef/LConn1
  Simulink-PS Converter/RConn1 -- Torque Lag/LConn1
  PS-Simulink Converter/LConn1 -- PS Product/RConn1
  PS Product/LConn1 -- PMSM/RConn2
  Power Sensor/LConn1 -- V/RConn1
  Power Sensor/RConn1 -- PMSM/LConn1

== system Hybrid_Series/Rev Counter ==
  Gain : Gain  Gain=-1
  Ideal Rotational Motion Sensor : fl_lib/Mechanical/Mechanical Sensors/Ideal Rotational Motion Sensor  offset=0 rad
  Ideal Torque Sensor : fl_lib/Mechanical/Mechanical Sensors/Ideal Torque Sensor
  Mechanical Rotational Reference : fl_lib/Mechanical/Rotational Elements/Mechanical Rotational Reference
  PS-Simulink Converter : nesl_utility/PS-Simulink Converter  PhysicalDomain=network_engine_domain  SubClassName=ps_output  LeftPortType=input  RightPortType=output  PseudoPeriodic=off  Frequencies=[]  Unit=rpm  AffineConversion=off
  PS-Simulink Converter1 : nesl_utility/PS-Simulink Converter  PhysicalDomain=network_engine_domain  SubClassName=ps_output  LeftPortType=input  RightPortType=output  PseudoPeriodic=off  Frequencies=[]  Unit=N*m  AffineConversion=off
  A : PMIOPort  Port=1  Side=Left
  B : PMIOPort  Port=2  Side=Left
  tag scope: Carrier_Trq_Nm=global, EngSpd_RPM=global
  wires:
  PS-Simulink Converter/1 -> [EngSpd_RPM]
  PS-Simulink Converter1/1 -> Gain/1
  Gain/1 -> [Carrier_Trq_Nm]
  connections:
  PS-Simulink Converter/LConn1 -- Ideal Rotational Motion Sensor/RConn2
  Mechanical Rotational Reference/LConn1 -- Ideal Rotational Motion Sensor/RConn1
  Ideal Rotational Motion Sensor/LConn1 -- A/RConn1 -- Ideal Torque Sensor/LConn1
  Ideal Torque Sensor/RConn2 -- PS-Simulink Converter1/LConn1
  B/RConn1 -- Ideal Torque Sensor/RConn1

== system Hybrid_Series/Routing ==
  M : Inport
  E : Inport  Port=2
  G : Inport  Port=3
  tag scope: ref_engine_speed=global, ref_generator_torque=global, ref_motor_rpm=global
  wires:
  E/1 -> [ref_engine_speed]
  G/1 -> [ref_generator_torque]
  M/1 -> [ref_motor_rpm]

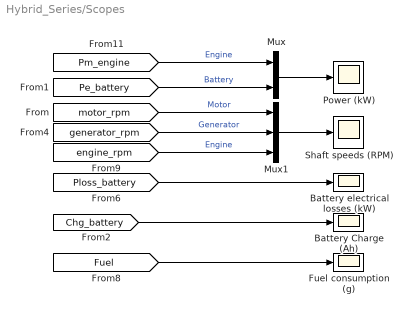
== system Hybrid_Series/Scopes ==
  Battery Charge (Ah) : Scope
  Battery electrical losses (kW) : Scope
  Fuel consumption (g) : Scope
  Mux : Mux  Inputs=2
  Mux1 : Mux  Inputs=3
  Power (kW) : Scope
  Shaft speeds (RPM) : Scope
  wires:
  Mux/1 -> Power (kW)/1
  Mux1/1 -> Shaft speeds (RPM)/1
  [motor_rpm] -> Mux1/1  "Motor"
  [generator_rpm] -> Mux1/2  "Generator"
  [engine_rpm] -> Mux1/3  "Engine"
  [Pm_engine] -> Mux/1  "Engine"
  [Pe_battery] -> Mux/2  "Battery"
  [Ploss_battery] -> Battery electrical losses (kW)/1
  [Fuel] -> Fuel consumption (g)/1
  [Chg_battery] -> Battery Charge (Ah)/1

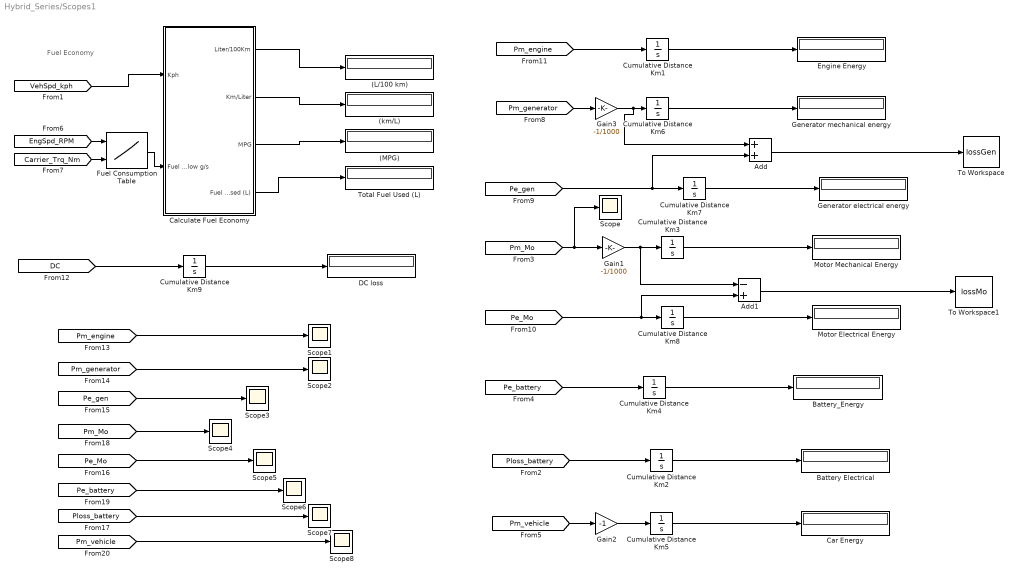
== system Hybrid_Series/Scopes1 ==
  note: Fuel Economy
  (L/100 km) : Display
      settings: Decimation=decimation
  (MPG) : Display
      settings: Decimation=decimation
  (km/L) : Display
      settings: Decimation=decimation
  Add : Sum
  Add1 : Sum  Inputs=-+
  Battery Electrical : Display
      settings: Decimation=decimation
  Battery_Energy : Display
      settings: Decimation=decimation
  Calculate Fuel Economy : Subsystem
  Car Energy : Display
      settings: Decimation=decimation
  Cumulative Distance Km{1..9} (9 alike) : Integrator  InitialCondition=eps
  DC loss : Display
      settings: Decimation=decimation
  Engine Energy : Display
      settings: Decimation=decimation
  Fuel Consumption Table : Lookup2D  RowIndex=HEV_Param.ICE.FC.Speed_Vector  ColumnIndex=HEV_Param.ICE.FC.Torque_Vector  Table=HEV_Param.ICE.FC.Consumption_Table
  Gain1 : Gain  Gain=-1/1000
  Gain2 : Gain  Gain=-1
  Gain3 : Gain  Gain=-1/1000
  Generator electrical energy : Display
      settings: Decimation=decimation
  Generator mechanical energy : Display
      settings: Decimation=decimation
  Motor Electrical Energy : Display
      settings: Decimation=decimation
  Motor Mechanical Energy : Display
      settings: Decimation=decimation
  Scope{,1..8} (9 alike) : Scope
  To Workspace : ToWorkspace  VariableName=lossGen  SampleTime=-1
      settings: Save2DSignal=2-D array (concatenate along first dimension)
  To Workspace1 : ToWorkspace  VariableName=lossMo  SampleTime=-1
      settings: Save2DSignal=2-D array (concatenate along first dimension)
  Total Fuel Used (L) : Display
      settings: Decimation=decimation
  wires:
  Cumulative Distance Km2/1 -> Battery Electrical/1
  [Ploss_battery] -> Cumulative Distance Km2/1
  Fuel Consumption Table/1 -> Calculate Fuel Economy/2(Fuel Flow g/s)
  Cumulative Distance Km5/1 -> Car Energy/1
  Gain2/1 -> Cumulative Distance Km5/1
  Cumulative Distance Km1/1 -> Engine Energy/1
  [Pm_engine] -> Cumulative Distance Km1/1
  Calculate Fuel Economy/1(Liter/100Km) -> (L/100 km)/1
  [VehSpd_kph] -> Calculate Fuel Economy/1(Kph)
  [Pe_battery] -> Cumulative Distance Km4/1
  [EngSpd_RPM] -> Fuel Consumption Table/1
  [Pm_Mo] -> Scope/1, Gain1/1
  Calculate Fuel Economy/3(MPG) -> (MPG)/1
  Cumulative Distance Km3/1 -> Motor Mechanical Energy/1
  [Carrier_Trq_Nm] -> Fuel Consumption Table/2
  Cumulative Distance Km4/1 -> Battery_Energy/1
  Calculate Fuel Economy/2(Km/Liter) -> (km/L)/1
  Calculate Fuel Economy/4(Fuel Used (L)) -> Total Fuel Used (L)/1
  [Pm_vehicle] -> Gain2/1
  Cumulative Distance Km6/1 -> Generator mechanical energy/1
  [Pm_generator] -> Gain3/1
  Gain3/1 -> Add/1, Cumulative Distance Km6/1
  [Pe_gen] -> Add/2, Cumulative Distance Km7/1
  Cumulative Distance Km7/1 -> Generator electrical energy/1
  Add/1 -> To Workspace/1
  Cumulative Distance Km8/1 -> Motor Electrical Energy/1
  Add1/1 -> To Workspace1/1
  [Pe_Mo] -> Add1/2, Cumulative Distance Km8/1
  Gain1/1 -> Add1/1, Cumulative Distance Km3/1
  Cumulative Distance Km9/1 -> DC loss/1
  [DC] -> Cumulative Distance Km9/1
  [Pm_engine] -> Scope1/1
  [Pm_generator] -> Scope2/1
  [Pe_gen] -> Scope3/1
  [Pm_Mo] -> Scope4/1
  [Pe_Mo] -> Scope5/1
  [Pe_battery] -> Scope6/1
  [Ploss_battery] -> Scope7/1
  [Pm_vehicle] -> Scope8/1

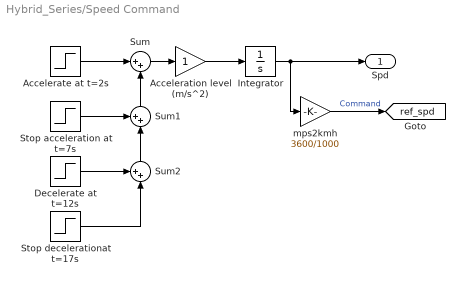
== system Hybrid_Series/Speed Command ==
  Accelerate at t=2s : Step  Time=2  SampleTime=0
  Acceleration level (m/s^2) : Gain
  Decelerate at t=12s : Step  Time=12  After=-1  SampleTime=0
  Integrator : Integrator  InitialCondition=v0
  Stop acceleration at t=7s : Step  Time=7  After=-1  SampleTime=0
  Stop decelerationat t=17s : Step  Time=17  SampleTime=0
  Sum : Sum  Inputs=|++
  Sum1 : Sum  Inputs=++|
  Sum2 : Sum  Inputs=++|
  mps2kmh : Gain  Gain=3600/1000
  Spd : Outport
  tag scope: ref_spd=global
  wires:
  mps2kmh/1 -> [ref_spd]  "Command"
  Stop decelerationat t=17s/1 -> Sum2/2
  Decelerate at t=12s/1 -> Sum2/1
  Acceleration level (m/s^2)/1 -> Integrator/1
  Sum2/1 -> Sum1/2
  Sum1/1 -> Sum/2
  Stop acceleration at t=7s/1 -> Sum1/1
  Integrator/1 -> Spd/1, mps2kmh/1
  Sum/1 -> Acceleration level (m/s^2)/1
  Accelerate at t=2s/1 -> Sum/1

== system Hybrid_Series/Strategy ==
  note: Generator torque demand has been set so that at the starting condition
      | the combustion engine is providing just enough power to keep the vehicle
      | moving at constant speed, and hence battery power is close to zero. The
      | engine RPM demand is set to 2000 rpm for good efficiency.
  Spd : Inport
  Convert to wheel RPM : Gain  Gain=60/(2*pi)/wheel_radius
  Engine RPM demand : Constant  Value=rpm0
  Generator torque demand : Constant  Value=-11
  Steady-state correction factor as proportional-only control : Gain  Gain=1.08
  Motor : Outport
  Engine : Outport  Port=2
  Gen : Outport  Port=3
  wires:
  Engine RPM demand/1 -> Steady-state correction factor as proportional-only control/1
  Spd/1 -> Convert to wheel RPM/1
  Convert to wheel RPM/1 -> Motor/1
  Steady-state correction factor as proportional-only control/1 -> Engine/1
  Generator torque demand/1 -> Gen/1

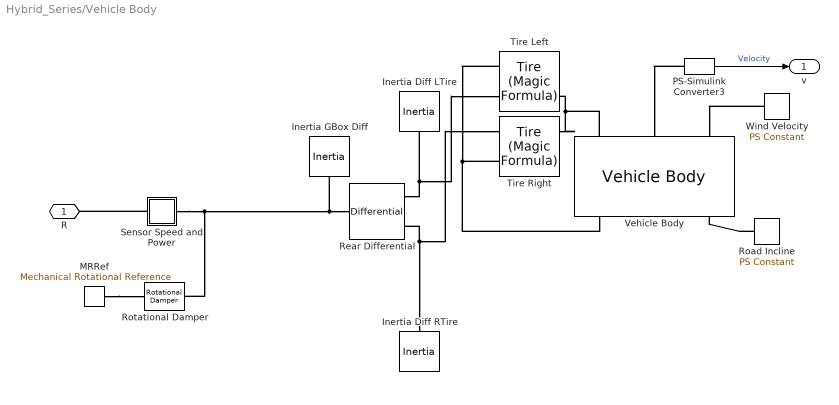
== system Hybrid_Series/Vehicle Body ==
  Inertia Diff LTire : fl_lib/Mechanical/Rotational Elements/Inertia  inertia=HEV_Param.Vehicle.Wheel_Inertia*2 kg*m^2  w_specify=on  w_priority=High  w=v0/wheel_radius rad/s  w_nominal_specify=off  w_nominal_unit=rad/s  w_nominal_value=1  t_specify=off  t_priority=High  t=0 N*m  t_nominal_specify=off  t_nominal_unit=N*m  t_nominal_value=1
  Inertia Diff RTire : fl_lib/Mechanical/Rotational Elements/Inertia  inertia=HEV_Param.Vehicle.Wheel_Inertia*2 kg*m^2  w_specify=on  w_priority=High  w=v0/wheel_radius rad/s  w_nominal_specify=off  w_nominal_unit=rad/s  w_nominal_value=1  t_specify=off  t_priority=High  t=0 N*m  t_nominal_specify=off  t_nominal_unit=N*m  t_nominal_value=1
  Inertia GBox Diff : fl_lib/Mechanical/Rotational Elements/Inertia  inertia=HEV_Param.Vehicle.Trans.Inertia kg*m^2  w_specify=on  w_priority=High  w=v0/wheel_radius rad/s  w_nominal_specify=off  w_nominal_unit=rad/s  w_nominal_value=1  t_specify=off  t_priority=High  t=0 N*m  t_nominal_specify=off  t_nominal_unit=N*m  t_nominal_value=1
  MRRef : fl_lib/Mechanical/Rotational Elements/Mechanical Rotational Reference
  PS-Simulink Converter3 : nesl_utility/PS-Simulink Converter  PhysicalDomain=network_engine_domain  SubClassName=ps_output  LeftPortType=input  RightPortType=output  PseudoPeriodic=off  Frequencies=[]  Unit=km/hr  AffineConversion=off
  Rear Differential : sdl_lib/Gears/Differential  driveshaft_location=2  cd_ratio=1  friction_model=1  efficiency=[ 0.85 0.92 ]  mu_visc=[ 0 0 ] N*m/(rad/s)  pwr_thr=[ 0.001 0.001 ] W  carrier_inertia=0 kg*m^2  planet_inertia=0 kg*m^2  temperature_TLU=[ 280 300 320 ] K  efficiency_ss_TLU=[ 0.95 0.9 0.85 ]  efficiency_cd_TLU=[ 0.95 0.9 0.85 ]  thermal_mass=50 J/K  T_init=300 K
      settings: SourceProductName=Simscape Driveline  SourceProductBaseCode=LD
  Road Incline : fl_lib/Physical Signals/Sources/PS Constant  constant=0
  Rotational Damper : fl_lib/Mechanical/Rotational Elements/Rotational Damper  D=HEV_Param.Vehicle.Trans.Friction N*m/(rad/s)  w_specify=on  w_priority=High  w=v0/wheel_radius rad/s  w_nominal_specify=off  w_nominal_unit=rad/s  w_nominal_value=1  t_specify=off  t_priority=High  t=0 N*m  t_nominal_specify=off  t_nominal_unit=N*m  t_nominal_value=1
  Sensor Speed and Power : Subsystem
      mask Display: disp('S')
  Tire Left : sdl_lib/Tires & Vehicles/Tire (Magic Formula)  parameterization=1  F_z1=HEV_Param.Vehicle.Tire.Rated_Vertical_Load N  F_x1=HEV_Param.Vehicle.Tire.Rated_Peak_Long_Force N  kappa1=HEV_Param.Vehicle.Tire.Slip_At_Peak_Force  B_m=10  C_m=1.9  D_m=1  E_m=0.97  fz0=4e+3 N  p_Cx=1.685  p_Dx=[ 1.21 -0.037 ]  p_Ex=[ 0.344 0.095 -0.02 0 ]  p_Kx=[ 21.51 -0.163 0.245 ]  p_Hx=[ -0.002 0.002 ]  p_Vx=[ 0 0 ]  v_tr_thr=0.1 m/s  r_e=HEV_Param.Vehicle.Tire_Radius m  model_compliance=0  stiffness=1e+6 N/m  damping=1000 N/(m/s)  model_inertia=1  inertia=1e-2 kg*m^2  initial_velocity=v0/wheel_radius rad/s  model_resistance=0  resistance_model=1  coeff=0.015  p_tire=2.5e+5 Pa  alpha=-0.003  beta=0.97  coeff_a=0.008399999999999999  coeff_b=6.2e-4 s/m  coeff_c=1.6e-4 s^2/m^2  v_thr=0.001 m/s
      settings: SourceProductName=Simscape Driveline
  Tire Right : sdl_lib/Tires & Vehicles/Tire (Magic Formula)  parameterization=1  F_z1=HEV_Param.Vehicle.Tire.Rated_Vertical_Load N  F_x1=HEV_Param.Vehicle.Tire.Rated_Peak_Long_Force N  kappa1=HEV_Param.Vehicle.Tire.Slip_At_Peak_Force  B_m=10  C_m=1.9  D_m=1  E_m=0.97  fz0=4e+3 N  p_Cx=1.685  p_Dx=[ 1.21 -0.037 ]  p_Ex=[ 0.344 0.095 -0.02 0 ]  p_Kx=[ 21.51 -0.163 0.245 ]  p_Hx=[ -0.002 0.002 ]  p_Vx=[ 0 0 ]  v_tr_thr=0.1 m/s  r_e=wheel_radius m  model_compliance=0  stiffness=1e+6 N/m  damping=1000 N/(m/s)  model_inertia=1  inertia=1e-2 kg*m^2  initial_velocity=v0/wheel_radius rad/s  model_resistance=0  resistance_model=1  coeff=0.015  p_tire=2.5e+5 Pa  alpha=-0.003  beta=0.97  coeff_a=0.008399999999999999  coeff_b=6.2e-4 s/m  coeff_c=1.6e-4 s^2/m^2  v_thr=0.001 m/s
      settings: SourceProductName=Simscape Driveline
  Vehicle Body : sdl_lib/Tires & Vehicles/Vehicle Body  mass=HEV_Param.Vehicle.Mass kg  n_w=2  x_f=HEV_Param.Vehicle.Distance_CG_FrontAxle m  x_r=HEV_Param.Vehicle.Distance_CG_RearAxle m  y_c=HEV_Param.Vehicle.Distance_CG_Ground m  area=HEV_Param.Vehicle.Frontal_Area m^2  Cd=HEV_Param.Vehicle.Aero_Drag_Coeff  g=9.81 m/s^2  rho=1.18 kg/m^3  v_specify=on  v_priority=High  v=v0 m/s  v_nominal_specify=off  v_nominal_unit=m/s  v_nominal_value=1
      settings: SourceProductName=Simscape Driveline
  Wind Velocity : fl_lib/Physical Signals/Sources/PS Constant  constant=0
  R : PMIOPort  Port=1  Side=Left
  v : Outport
  wires:
  PS-Simulink Converter3/1 -> v/1  "Velocity"
  connections:
  Vehicle Body/RConn1 -- Tire Right/LConn1 -- Tire Left/LConn1
  Vehicle Body/LConn1 -- Tire Right/RConn2 -- Tire Left/RConn2
  PS-Simulink Converter3/LConn1 -- Vehicle Body/LConn2
  Road Incline/RConn1 -- Vehicle Body/RConn3
  Wind Velocity/RConn1 -- Vehicle Body/LConn3
  Rear Differential/RConn1 -- Tire Right/LConn2 -- Inertia Diff RTire/LConn1
  Rear Differential/RConn2 -- Tire Left/LConn2 -- Inertia Diff LTire/LConn1
  Sensor Speed and Power/RConn1 -- Inertia GBox Diff/LConn1 -- Rear Differential/LConn1 -- Rotational Damper/LConn1
  Sensor Speed and Power/LConn1 -- R/RConn1
  MRRef/LConn1 -- Rotational Damper/RConn1

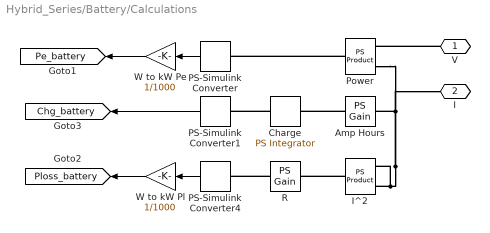
== system Hybrid_Series/Battery/Calculations ==
  " W to kW Pe" : Gain  Gain=1/1000
  " W to kW Pl " : Gain  Gain=1/1000
  Amp Hours : fl_lib/Physical Signals/Functions/PS Gain  gain=-1/(60*60)
  Charge : fl_lib/Physical Signals/Linear Operators/PS Integrator  x0=150
      settings: SourceProductName=Simscape  SourceProductBaseCode=SS
  I^2 : fl_lib/Physical Signals/Functions/PS Product
      settings: SourceProductName=Simscape
  PS-Simulink Converter : nesl_utility/PS-Simulink Converter  PhysicalDomain=network_engine_domain  SubClassName=ps_output  LeftPortType=input  RightPortType=output  PseudoPeriodic=off  Frequencies=[]  Unit=kW  AffineConversion=off
  PS-Simulink Converter1 : nesl_utility/PS-Simulink Converter  PhysicalDomain=network_engine_domain  SubClassName=ps_output  LeftPortType=input  RightPortType=output  PseudoPeriodic=off  Frequencies=[]  Unit=1  AffineConversion=off
  PS-Simulink Converter4 : nesl_utility/PS-Simulink Converter  PhysicalDomain=network_engine_domain  SubClassName=ps_output  LeftPortType=input  RightPortType=output  PseudoPeriodic=off  Frequencies=[]  Unit=1  AffineConversion=off
  Power : fl_lib/Physical Signals/Functions/PS Product
      settings: SourceProductName=Simscape
  R : fl_lib/Physical Signals/Functions/PS Gain  gain=0.05
  V : PMIOPort  Port=1  Side=Left
  I : PMIOPort  Port=2  Side=Left
  tag scope: Chg_battery=global, Pe_battery=global, Ploss_battery=global
  wires:
  " W to kW Pl "/1 -> [Ploss_battery]
  PS-Simulink Converter4/1 -> " W to kW Pl "/1
  PS-Simulink Converter1/1 -> [Chg_battery]
  PS-Simulink Converter/1 -> " W to kW Pe"/1
  " W to kW Pe"/1 -> [Pe_battery]
  connections:
  R/RConn1 -- PS-Simulink Converter4/LConn1
  I^2/RConn1 -- R/LConn1
  Amp Hours/RConn1 -- Charge/LConn1
  I^2/LConn2 -- I/RConn1 -- Power/LConn2 -- Amp Hours/LConn1 -- I^2/LConn1
  V/RConn1 -- Power/LConn1
  Power/RConn1 -- PS-Simulink Converter/LConn1
  Charge/RConn1 -- PS-Simulink Converter1/LConn1

== system Hybrid_Series/DC Converter/Control Bus Voltage ==
  Ki : fl_lib/Physical Signals/Functions/PS Gain  gain=Ki
  Kp : fl_lib/Physical Signals/Functions/PS Gain  gain=Kp
  PS Add1 : fl_lib/Physical Signals/Functions/PS Add
  PS Integrator : fl_lib/Physical Signals/Linear Operators/PS Integrator  x0=Vout
      settings: SourceProductName=Simscape  SourceProductBaseCode=SS
  PS Subtract : fl_lib/Physical Signals/Functions/PS Subtract
      settings: SourceProductName=Simscape
  Vmeas : PMIOPort  Port=1  Side=Left
  Vref : PMIOPort  Port=2  Side=Left
  VBus : PMIOPort  Port=3  Side=Right
  connections:
  PS Integrator/RConn1 -- PS Add1/LConn1
  PS Add1/LConn2 -- Kp/RConn1
  Kp/LConn1 -- PS Subtract/RConn1 -- Ki/LConn1
  PS Integrator/LConn1 -- Ki/RConn1
  Vmeas/RConn1 -- PS Subtract/LConn2
  Vref/RConn1 -- PS Subtract/LConn1
  VBus/RConn1 -- PS Add1/RConn1

== system Hybrid_Series/DC Converter/Current Sensor ==
  Current Sensor : fl_lib/Electrical/Electrical Sensors/Current Sensor
  PS-Simulink Converter : nesl_utility/PS-Simulink Converter  PhysicalDomain=network_engine_domain  SubClassName=ps_output  LeftPortType=input  RightPortType=output  PseudoPeriodic=off  Frequencies=[]  Unit=1  AffineConversion=off
  I : PMIOPort  Port=1  Side=Right
  + : PMIOPort  Port=2  Side=Left
  - : PMIOPort  Port=3  Side=Right
  tag scope: I_out=global
  wires:
  PS-Simulink Converter/1 -> [I_out]
  connections:
  -/RConn1 -- Current Sensor/RConn2
  +/RConn1 -- Current Sensor/LConn1
  PS-Simulink Converter/LConn1 -- I/RConn1 -- Current Sensor/RConn1

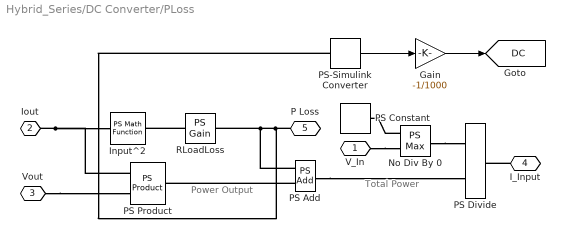
== system Hybrid_Series/DC Converter/PLoss ==
  note: Total Power
  note: Power Output
  Gain : Gain  Gain=-1/1000
  Input^2 : fl_lib/Physical Signals/Functions/PS Math Function  fcn_choice=7
      settings: SourceProductName=Simscape  SourceProductBaseCode=SS
  No Div By 0 : fl_lib/Physical Signals/Nonlinear Operators/PS Max
      settings: SourceProductName=Simscape  SourceProductBaseCode=SS
  PS Add : fl_lib/Physical Signals/Functions/PS Add
  PS Constant : fl_lib/Physical Signals/Sources/PS Constant  constant=HEV_Param.DCDCConv.MinVin
  PS Divide : fl_lib/Physical Signals/Functions/PS Divide
      settings: SourceProductName=Simscape  SourceProductBaseCode=SS
  PS Product : fl_lib/Physical Signals/Functions/PS Product
      settings: SourceProductName=Simscape
  PS-Simulink Converter : nesl_utility/PS-Simulink Converter  PhysicalDomain=network_engine_domain  SubClassName=ps_output  LeftPortType=input  RightPortType=output  PseudoPeriodic=off  Frequencies=[]  Unit=1  AffineConversion=off
  RLoadLoss : fl_lib/Physical Signals/Functions/PS Gain  gain=RLoadLoss
  V_In : PMIOPort  Port=1  Side=Left
  Iout : PMIOPort  Port=2  Side=Left
  Vout : PMIOPort  Port=3  Side=Left
  I_Input : PMIOPort  Port=4  Side=Right
  P Loss : PMIOPort  Port=5  Side=Right
  tag scope: DC=global
  wires:
  Gain/1 -> [DC]
  PS-Simulink Converter/1 -> Gain/1
  connections:
  PS Add/RConn1 -- PS Divide/LConn1
  No Div By 0/RConn1 -- PS Divide/LConn2
  V_In/RConn1 -- No Div By 0/LConn2
  No Div By 0/LConn1 -- PS Constant/RConn1
  P Loss/RConn1 -- RLoadLoss/RConn1 -- PS Add/LConn1 -- PS-Simulink Converter/LConn1
  PS Add/LConn2 -- PS Product/RConn1
  RLoadLoss/LConn1 -- Input^2/RConn1
  Iout/RConn1 -- PS Product/LConn1 -- Input^2/LConn1
  Vout/RConn1 -- PS Product/LConn2
  I_Input/RConn1 -- PS Divide/RConn1

== system Hybrid_Series/DC Converter/Subsystem3 ==
  Out : PMIOPort  Tag=PMCPort  Port=1  Side=Right
  In : PMIOPort  Tag=PMCPort  Port=2  Side=Left
  connections:
  In/RConn1 -- Out/RConn1
